simulink model "Tiny"  (R2017b)
settings: Solver=ode3  StartTime=0.0  StopTime=SimTime  FixedStep=0.1  RelTol=1e-3  EnableMultiTasking=on
settings Model: Creator=aarrieta  LastModifiedBy=ainhoaarruabarrenaortiz
settings DataIOCC: LimitDataPoints=on  SaveFormat=Array
settings OptimizationCC: LifeSpan=inf
settings DebuggingCC: UnderspecifiedInitializationDetection=Classic  MergeDetectMultiDrivingBlocksExec=none  SolverPrmCheckMsg=warning  StateNameClashWarn=warning  SFUnexpectedBacktrackingDiag=warning  SFNoUnconditionalDefaultTransitionDiag=warning  SFExecutionAtInitializationDiag=none
settings HardwareCC: ProdBitPerPointer=32  ProdBitPerSizeT=32  ProdBitPerPtrDiffT=32  ProdLargestAtomicFloat=None  ProdIntDivRoundTo=Undefined  ProdEndianess=Unspecified  ProdWordSize=32  ProdHWDeviceType=32-bit Generic
settings ModelReferenceCC: PropagateSignalLabelsOutOfModel=off
settings CodeAppCC: StateflowObjectComments=on
settings GRTTargetCC: TargetLangStandard=C89/C90 (ANSI)  GeneratePreprocessorConditionals=Disable all
settings ConfigComp: CovMetricSettings=dw  CovHtmlReporting=on  CovSaveCumulativeToWorkspaceVar=on  CovSaveSingleToWorkspaceVar=on  CovExternalEMLEnable=off

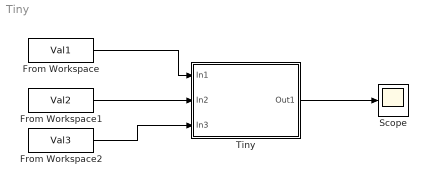
== system Tiny ==
  From Workspace : FromWorkspace  VariableName=Val1  SampleTime=0
  From Workspace1 : FromWorkspace  VariableName=Val2  SampleTime=0
  From Workspace2 : FromWorkspace  VariableName=Val3  SampleTime=0
  Scope : Scope
  Tiny : Subsystem
  wires:
  From Workspace2/1 -> Tiny/3(In3)
  From Workspace1/1 -> Tiny/2(In2)
  From Workspace/1 -> Tiny/1(In1)
  Tiny/1(Out1) -> Scope/1

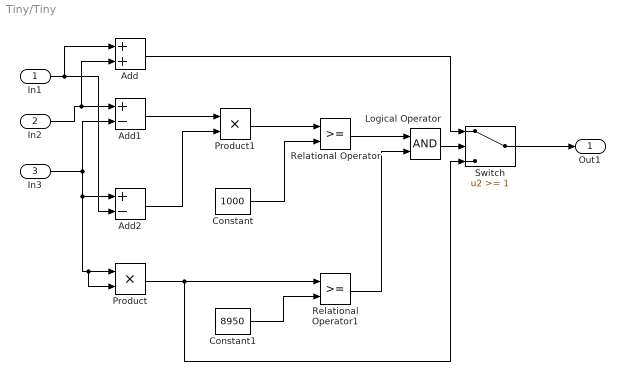
== system Tiny/Tiny ==
  In1 : Inport
  In2 : Inport  Port=2
  In3 : Inport  Port=3
  Add : Sum
  Add1 : Sum  Inputs=+-
  Add2 : Sum  Inputs=+-
  Constant : Constant  Value=1000
  Constant1 : Constant  Value=8950
  Logical Operator : Logic  AllPortsSameDT=off  OutDataTypeStr=boolean
  Product : Product
  Product1 : Product
  Relational Operator : RelationalOperator  OutDataTypeStr=boolean  RndMeth=Nearest
  Relational Operator1 : RelationalOperator  OutDataTypeStr=boolean  RndMeth=Nearest
  Switch : Switch  Threshold=1
  Out1 : Outport
  wires:
  In3/1 -> Add2/1, Product/2, Product/1, Add1/2
  In1/1 -> Add/1, Add2/2
  In2/1 -> Add/2, Add1/1
  Add1/1 -> Product1/1
  Add2/1 -> Product1/2
  Product1/1 -> Relational Operator/1
  Product/1 -> Switch/3, Relational Operator1/1
  Constant/1 -> Relational Operator/2
  Constant1/1 -> Relational Operator1/2
  Relational Operator/1 -> Logical Operator/1
  Relational Operator1/1 -> Logical Operator/2
  Logical Operator/1 -> Switch/2
  Add/1 -> Switch/1
  Switch/1 -> Out1/1
